simulink model "ModelWithApproximation_20210824T102023489"  (R2020a)
settings: Solver=FixedStepAuto  StartTime=0.0  StopTime=size(InputValues_20210824T100641914,1) - 1  FixedStep=1  RelTol=1e-3
model workspace (MAT data in the model file):
  InputValues_20210824T100641914 = [-5; -4.9375; -4.875; -4.8125; -4.75; -4.6875; -4.625; -4.5625; -4.5; -4.4375; -4.375; -4.3125; -4.25; -4.1875; -4.125; -4.0625; -4; -3.9375; -3.875; -3.8125; -3.75; -3.6875; -3.625; -3.5625; -3.5; -3.4375; -3.375; -3.3125; -3.25; -3.1875; -3.125; -3.0625; -3; -2.9375; -2.875; -2.8125; -2.75; -2.6875; -2.625; -2.5625; -2.5; -2.4375; -2.375; -2.3125; -2.25; -2.1875; -2.125; -2.0625; -2; -1.9375; -1.875; -1.8125; -1.75; -1.6875; -1.625; -1.5625; -1.5; -1.4375; -1.375; -1.3125; -1.25; -1.1875; -1.125; -1.0625; -1; -0.9375; -0.875; -0.8125; -0.75; -0.6875; -0.625; -0.5625; -0.5; -0.4375; -0.375; -0.3125; -0.25; -0.1875; -0.125; -0.0625; 0; 0.0625; 0.125; 0.1875; 0.25; 0.3125; 0.375; 0.4375; 0.5; 0.5625; 0.625; 0.6875; 0.75; 0.8125; 0.875; 0.9375; 1; 1.0625; 1.125; 1.1875; 1.25; 1.3125; 1.375; 1.4375; 1.5; 1.5625; 1.625; 1.6875; 1.75; 1.8125; 1.875; 1.9375; 2; 2.0625; 2.125; 2.1875; 2.25; 2.3125; 2.375; 2.4375; 2.5; 2.5625; 2.625; 2.6875; 2.75; 2.8125; 2.875; 2.9375; 3; 3.0625; 3.125; 3.1875; 3.25; 3.3125; 3.375; 3.4375; 3.5; 3.5625; 3.625; 3.6875; 3.75; 3.8125; 3.875; 3.9375; 4; 4.0625; 4.125; 4.1875; 4.25; 4.3125; 4.375; 4.4375; 4.5; 4.5625; 4.625; 4.6875; 4.75; 4.8125; 4.875; 4.9375; 5]
undefined symbols (not defined in the file or in its folder): FunctionApproximation
libraries: simulink x1
settings Model: OrderedModelArguments=off  Creator=Mahsa  LastModifiedBy=Mahsa
settings DebuggingCC: IntegerOverflowMsg=none  ParameterOverflowMsg=none  ParameterPrecisionLossMsg=none  IntegerSaturationMsg=none

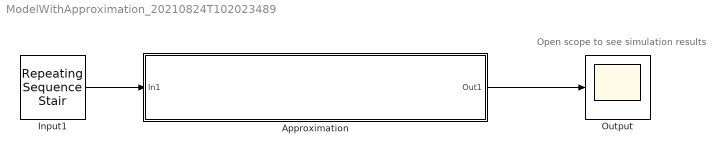
== system ModelWithApproximation_20210824T102023489 ==
  note: Open scope to see simulation results
  Approximation : Subsystem  Description=This block was created using function approximation.  Variant=on  mask(Function Approximation Solution){variantTag=3112e06394ab71adacf7bb189cb322dbc695f0e4, createdBy=FunctionApproximation, currentActive=Approximate, nApproximates=1, createdOn=20210824T102019933, matlabVersion={"Name":"MATLAB","Version":"9.8","Release":"(R2020a)","Date":"18-Nov-2019"}, functionVersion=Approximate, problemStruct={"FunctionToApproximate":"@(x)tanh(x)","InputTypes":"numerictype(1,8,4)","InputLowerBounds":"-5","InputUpperBounds":"5","OutputType":"numerictype(1,8,7)","Options":{"WordLengths":"[8]","BreakpointSpecification":"EvenPow2Spacing","AbsTol":"0.0078125","RelTol":"0.0078125","AllowUpdateDiagram":"1","Display":"0","Interpolation":"Flat","SaturateToOutputType":"1","MaxTime":"Inf","MaxMemoryUsage":"80000000","MemoryUnits":"bits","OnCurveTableValues":"0","AUTOSARCompliant":"0","UseParallel":"0"},"FunctionToReplace":"","InputFunctionType":"SpecialFunctionHandle","StorageTypes":[],"DependentVariables":[]}, compareData={"Breakpoints":[[-5,-4.9375,-4.875,-4.8125,-4.75,-4.6875,-4.625,-4.5625,-4.5,-4.4375,-4.375,-4.3125,-4.25,-4.1875,-4.125,-4.0625,-4,-3.9375,-3.875,-3.8125,-3.75,-3.6875,-3.625,-3.5625,-3.5,-3.4375,-3.375,-3.3125,-3.25,-3.1875,-3.125,-3.0625,-3,-2.9375,-2.875,-2.8125,-2.75,-2.6875,-2.625,-2.5625,-2.5,-2.4375,-2.375,-2.3125,-2.25,-2.1875,-2.125,-2.0625,-2,-1.9375,-1.875,-1.8125,-1.75,-1.6875,-1.625,-1.5625,-1.5,-1.4375,-1.375,-1.3125,-1.25,-1.1875,-1.125,-1.0625,-1,-0.9375,-0.875,-0.8125,-0.75,-0.6875,-0.625,-0.5625,-0.5,-0.4375,-0.375,-0.3125,-0.25,-0.1875,-0.125,-0.0625,0,0.0625,0.125,0.1875,0.25,0.3125,0.375,0.4375,0.5,0.5625,0.625,0.6875,0.75,0.8125,0.875,0.9375,1,1.0625,1.125,1.1875,1.25,1.3125,1.375,1.4375,1.5,1.5625,1.625,1.6875,1.75,1.8125,1.875,1.9375,2,2.0625,2.125,2.1875,2.25,2.3125,2.375,2.4375,2.5,2.5625,2.625,2.6875,2.75,2.8125,2.875,2.9375,3,3.0625,3.125,3.1875,3.25,3.3125,3.375,3.4375,3.5,3.5625,3.625,3.6875,3.75,3.8125,3.875,3.9375,4,4.0625,4.125,4.1875,4.25,4.3125,4.375,4.4375,4.5,4.5625,4.625,4.6875,4.75,4.8125,4.875,4.9375,5]],"Original":[-0.99990920426259511,-0.99989711557251559,-0.9998834174686777,-0.99986789571029067,-0.99985030754497872,-0.99983037791655283,-0.99980779516900109,-0.99978220617994684,-0.99975321084802748,-0.99972035584870533,-0.99968312756179489,-0.99964094406130644,-0.9995931460438896,-0.9995389865560137,-0.99947761936180857,-0.9994080857729738,-0.999329299739067,-0.9992400309704963,-0.99913888583735078,-0.99902428575443547,-0.9988944427261528,-0.99874733168378116,-0.99858065920179884,-0.9983918281287415,-0.99817789761119868,-0.99793553792649037,-0.997660979469889,-0.99734995516557368,-0.996997635486526,-0.99659855517712947,-0.996146530673345,-0.99563456710930964,-0.99505475368673046,-0.994398146065758,-0.99365463431502965,-0.99281279483715978,-0.9918597245682077,-0.99078085564125162,-0.98955974861288321,-0.98817786228751237,-0.98661429815143031,-0.9848455174642784,-0.982845029172576,-0.9805830470370519,-0.97802611473881362,-0.97513669829362837,-0.971872745913509,-0.96818721657637052,-0.9640275800758169,-0.95933529331468248,-0.95404526017994873,-0.9480852856044063,-0.94137553849728739,-0.93382804322259172,-0.925346225311741,-0.91582454416876236,-0.9051482536448664,-0.89319334040035159,-0.87982669965198479,-0.86490661772074184,-0.84828363995751288,-0.82980190998595948,-0.809301070201781,-0.78661881210869766,-0.76159415595576485,-0.73407151960434158,-0.70390560393662116,-0.67096707420687374,-0.6351489523872873,-0.59637355547924231,-0.55459972234938226,-0.50982997373525663,-0.46211715726000974,-0.41157005567402238,-0.35835739835078595,-0.30270972933210849,-0.24491866240370913,-0.18533319990813948,-0.12435300177159619,-0.062418746747512514,0,0.062418746747512514,0.12435300177159619,0.18533319990813948,0.24491866240370913,0.30270972933210849,0.35835739835078595,0.41157005567402238,0.46211715726000974,0.50982997373525663,0.55459972234938226,0.59637355547924231,0.6351489523872873,0.67096707420687374,0.70390560393662116,0.73407151960434158,0.76159415595576485,0.78661881210869766,0.809301070201781,0.82980190998595948,0.84828363995751288,0.86490661772074184,0.87982669965198479,0.89319334040035159,0.9051482536448664,0.91582454416876236,0.925346225311741,0.93382804322259172,0.94137553849728739,0.9480852856044063,0.95404526017994873,0.95933529331468248,0.9640275800758169,0.96818721657637052,0.971872745913509,0.97513669829362837,0.97802611473881362,0.9805830470370519,0.982845029172576,0.9848455174642784,0.98661429815143031,0.98817786228751237,0.98955974861288321,0.99078085564125162,0.9918597245682077,0.9921875,0.9921875,0.9921875,0.9921875,0.9921875,0.9921875,0.9921875,0.9921875,0.9921875,0.9921875,0.9921875,0.9921875,0.9921875,0.9921875,0.9921875,0.9921875,0.9921875,0.9921875,0.9921875,0.9921875,0.9921875,0.9921875,0.9921875,0.9921875,0.9921875,0.9921875,0.9921875,0.9921875,0.9921875,0.9921875,0.9921875,0.9921875,0.9921875,0.9921875,0.9921875,0.9921875],"Approximate":[-1,-1,-1,-1,-1,-1,-1,-1,-1,-1,-1,-1,-1,-1,-1,-1,-1,-1,-1,-1,-1,-1,-1,-1,-1,-1,-1,-1,-1,-1,-1,-0.9921875,-0.9921875,-0.9921875,-0.9921875,-0.9921875,-0.9921875,-0.9921875,-0.9921875,-0.984375,-0.984375,-0.984375,-0.984375,-0.984375,-0.9765625,-0.9765625,-0.96875,-0.96875,-0.9609375,-0.9609375,-0.953125,-0.9453125,-0.9375,-0.9375,-0.921875,-0.9140625,-0.90625,-0.890625,-0.8828125,-0.8671875,-0.8515625,-0.828125,-0.8125,-0.7890625,-0.7578125,-0.734375,-0.703125,-0.671875,-0.6328125,-0.59375,-0.5546875,-0.5078125,-0.4609375,-0.4140625,-0.359375,-0.3046875,-0.2421875,-0.1875,-0.125,-0.0625,0,0.0625,0.125,0.1875,0.2421875,0.3046875,0.359375,0.4140625,0.4609375,0.5078125,0.5546875,0.59375,0.6328125,0.671875,0.703125,0.734375,0.7578125,0.7890625,0.8125,0.828125,0.8515625,0.8671875,0.8828125,0.890625,0.90625,0.9140625,0.921875,0.9375,0.9375,0.9453125,0.953125,0.9609375,0.9609375,0.96875,0.96875,0.9765625,0.9765625,0.984375,0.984375,0.984375,0.984375,0.984375,0.9921875,0.9921875,0.9921875,0.9921875,0.9921875,0.9921875,0.9921875,0.9921875,0.9921875,0.9921875,0.9921875,0.9921875,0.9921875,0.9921875,0.9921875,0.9921875,0.9921875,0.9921875,0.9921875,0.9921875,0.9921875,0.9921875,0.9921875,0.9921875,0.9921875,0.9921875,0.9921875,0.9921875,0.9921875,0.9921875,0.9921875,0.9921875,0.9921875,0.9921875,0.9921875,0.9921875,0.9921875,0.9921875,0.9921875],"AbsDiff":[9.0795737404891774E-5,0.00010288442748440652,0.00011658253132229568,0.00013210428970933386,0.00014969245502127748,0.000169622083447174,0.00019220483099890995,0.00021779382005315817,0.00024678915197251516,0.0002796441512946668,0.00031687243820510691,0.00035905593869356434,0.00040685395611039787,0.00046101344398630228,0.0005223806381914331,0.00059191422702620233,0.000670700260932966,0.00075996902950370426,0.00086111416264922358,0.00097571424556452957,0.0011055572738472019,0.0012526683162188412,0.001419340798201163,0.0016081718712585014,0.0018221023888013166,0.002064462073509632,0.0023390205301110356,0.0026500448344263239,0.0030023645134740207,0.0034014448228705252,0.0038534693266549791,0.0034470671093096428,0.0028672536867304643,0.0022106460657580485,0.00146713431502965,0.0006252948371597844,0.00032777543179229873,0.0014066443587483768,0.0026277513871167946,0.0038028622875123652,0.0022392981514303134,0.00047051746427839714,0.0015299708274240098,0.0037919529629480975,0.0014636147388136234,0.0014258017063716322,0.0031227459135090285,0.000562783423629476,0.0030900800758169034,0.0016022066853175199,0.00092026017994872866,0.0027727856044063026,0.0038755384972873896,0.0036719567774082806,0.0034712253117410441,0.0017620441687623556,0.0011017463551336037,0.0025683404003515875,0.0029858003480152107,0.0022808822792581562,0.0032788600424871195,0.0016769099859594849,0.0031989297982190079,0.0024436878913023374,0.003781655955764851,0.00030348039565841756,0.00078060393662116034,0.000907925793126263,0.0023364523872873022,0.0026235554792423121,8.7777650617737457E-5,0.0020174737352566252,0.0011796572600097366,0.0024924443259776163,0.0010176016492140505,0.0019777706678915097,0.0027311624037091309,0.0021668000918605157,0.00064699822840380561,8.1253252487485661E-5,0,8.1253252487485661E-5,0.00064699822840380561,0.0021668000918605157,0.0027311624037091309,0.0019777706678915097,0.0010176016492140505,0.0024924443259776163,0.0011796572600097366,0.0020174737352566252,8.7777650617737457E-5,0.0026235554792423121,0.0023364523872873022,0.000907925793126263,0.00078060393662116034,0.00030348039565841756,0.003781655955764851,0.0024436878913023374,0.0031989297982190079,0.0016769099859594849,0.0032788600424871195,0.0022808822792581562,0.0029858003480152107,0.0025683404003515875,0.0011017463551336037,0.0017620441687623556,0.0034712253117410441,0.0036719567774082806,0.0038755384972873896,0.0027727856044063026,0.00092026017994872866,0.0016022066853175199,0.0030900800758169034,0.000562783423629476,0.0031227459135090285,0.0014258017063716322,0.0014636147388136234,0.0037919529629480975,0.0015299708274240098,0.00047051746427839714,0.0022392981514303134,0.0038028622875123652,0.0026277513871167946,0.0014066443587483768,0.00032777543179229873,0,0,0,0,0,0,0,0,0,0,0,0,0,0,0,0,0,0,0,0,0,0,0,0,0,0,0,0,0,0,0,0,0,0,0,0],"MaxDiff":[0.0078125,0.0078125,0.0078125,0.0078125,0.0078125,0.0078125,0.0078125,0.0078125,0.0078125,0.0078125,0.0078125,0.0078125,0.0078125,0.0078125,0.0078125,0.0078125,0.0078125,0.0078125,0.0078125,0.0078125,0.0078125,0.0078125,0.0078125,0.0078125,0.0078125,0.0078125,0.0078125,0.0078125,0.0078125,0.0078125,0.0078125,0.0078125,0.0078125,0.0078125,0.0078125,0.0078125,0.0078125,0.0078125,0.0078125,0.0078125,0.0078125,0.0078125,0.0078125,0.0078125,0.0078125,0.0078125,0.0078125,0.0078125,0.0078125,0.0078125,0.0078125,0.0078125,0.0078125,0.0078125,0.0078125,0.0078125,0.0078125,0.0078125,0.0078125,0.0078125,0.0078125,0.0078125,0.0078125,0.0078125,0.0078125,0.0078125,0.0078125,0.0078125,0.0078125,0.0078125,0.0078125,0.0078125,0.0078125,0.0078125,0.0078125,0.0078125,0.0078125,0.0078125,0.0078125,0.0078125,0.0078125,0.0078125,0.0078125,0.0078125,0.0078125,0.0078125,0.0078125,0.0078125,0.0078125,0.0078125,0.0078125,0.0078125,0.0078125,0.0078125,0.0078125,0.0078125,0.0078125,0.0078125,0.0078125,0.0078125,0.0078125,0.0078125,0.0078125,0.0078125,0.0078125,0.0078125,0.0078125,0.0078125,0.0078125,0.0078125,0.0078125,0.0078125,0.0078125,0.0078125,0.0078125,0.0078125,0.0078125,0.0078125,0.0078125,0.0078125,0.0078125,0.0078125,0.0078125,0.0078125,0.0078125,0.0078125,0.0078125,0.0078125,0.0078125,0.0078125,0.0078125,0.0078125,0.0078125,0.0078125,0.0078125,0.0078125,0.0078125,0.0078125,0.0078125,0.0078125,0.0078125,0.0078125,0.0078125,0.0078125,0.0078125,0.0078125,0.0078125,0.0078125,0.0078125,0.0078125,0.0078125,0.0078125,0.0078125,0.0078125,0.0078125,0.0078125,0.0078125,0.0078125,0.0078125,0.0078125,0.0078125],"Feasible":true,"Options":{"WordLengths":8,"BreakpointSpecification":"EvenPow2Spacing","AbsTol":0.0078125,"RelTol":0.0078125,"AllowUpdateDiagram":true,"Display":true,"Interpolation":"Flat","SaturateToOutputType":true,"MaxTime":null,"MaxMemoryUsage":8.0E+7,"MemoryUnits":"bits","OnCurveTableValues":false,"AUTOSARCompliant":false,"UseParallel":false}}}
      mask prompts: functionVersion "Select desired function version"
      mask help: This block contains the original and approximate functions.
      settings: CopyFcn=FunctionApproximation.internal.approximationblock.callback.updateTag('3112e06394ab71adacf7bb189cb322dbc695f0e4');  OpenFcn=FunctionApproximation.internal.approximationblock.callback.openMask('3112e06394ab71adacf7bb189cb322dbc695f0e4');
      mask Help: helpview(fullfile(docroot,'fixedpoint','fixedpoint.map'), 'function_approximation_block')
      mask TypeOptions functionVersion: Original | Approximate
      mask Callback functionVersion: FunctionApproximation.internal.approximationblock.callback.registerActiveFunction('3112e06394ab71adacf7bb189cb322dbc695f0e4');
      mask DialogControl details Prompt: Problem Definition
      mask DialogControl details Tooltip: Details of problem definition for approximation
      mask DialogControl detailsText Prompt:
      | Inputs for approximation:
      |   InputLowerBounds: -5
      |   InputTypes: numerictype(1,8,4)
      |   InputUpperBounds: 5
      |   OutputType: numerictype(1,8,7)
      |   Options (non-default)
      |     AbsTol: 0.0078125
      |     BreakpointSpecification: EvenPow2Spacing
      |     Display: 0
      |     Interpolation: Flat
      |     OnCurveTableValues: 0
      |     RelTol: 0.0078125
      |     SaturateToOutputType: 1
      |     WordLengths: [8]
      mask DialogControl showOriginal Prompt: Show original
      mask DialogControl showOriginal Tooltip: View the original function
      mask DialogControl showOriginal Callback: FunctionApproximation.internal.approximationblock.callback.showFunction('3112e06394ab71adacf7bb189cb322dbc695f0e4','Original');
      mask DialogControl showCurrent Prompt: Show selected
      mask DialogControl showCurrent Tooltip: View the selected function
      mask DialogControl showCurrent Callback: FunctionApproximation.internal.approximationblock.callback.showCurrent('3112e06394ab71adacf7bb189cb322dbc695f0e4');
      mask DialogControl revertToOriginal Prompt: Replace with original
      mask DialogControl revertToOriginal Tooltip: Replace current block with the original function
      mask DialogControl revertToOriginal Callback: FunctionApproximation.internal.approximationblock.callback.revertDialog('3112e06394ab71adacf7bb189cb322dbc695f0e4');
      mask DialogControl redesign Prompt: Redesign approximate
      mask DialogControl redesign Tooltip: Obtain a new approximate for the original function.
      mask DialogControl redesign Callback: FunctionApproximation.internal.approximationblock.callback.redesign('3112e06394ab71adacf7bb189cb322dbc695f0e4');
      mask DialogControl compare Prompt: Compare to original
      mask DialogControl compare Tooltip: Visualize difference between original and selected function.
      mask DialogControl compare Callback: FunctionApproximation.internal.approximationblock.callback.compareToOriginal('3112e06394ab71adacf7bb189cb322dbc695f0e4');
  Input1 : simulink/Sources/Repeating Sequence Stair  OutValues=InputValues_20210824T100641914(:,1)  tsamp=-1  OutMin=[]  OutMax=[]  OutDataTypeStr=double  OutputDataTypeScalingMode=double  OutDataType=fixdt(0,8)  ConRadixGroup=Best Precision: Vector-wise  OutScaling=2^-12
  Output : Scope
  wires:
  Input1/1 -> Approximation/1(In1)
  Approximation/1(Out1) -> Output/1

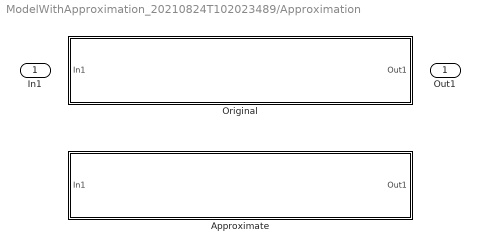
== system ModelWithApproximation_20210824T102023489/Approximation ==
  In1 : Inport
  Approximate : Subsystem  Tag=Approximate  VariantControl=FunctionApproximation.internal.approximationblock.callback.isCurrent('3112e06394ab71adacf7bb189cb322dbc695f0e4','Approximate')
  Original : Subsystem  Tag=Original  VariantControl=FunctionApproximation.internal.approximationblock.callback.isCurrent('3112e06394ab71adacf7bb189cb322dbc695f0e4','Original')
  Out1 : Outport

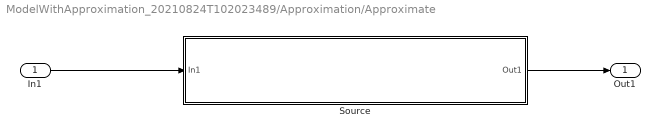
== system ModelWithApproximation_20210824T102023489/Approximation/Approximate ==
  In1 : Inport
  Source : Subsystem  Description=This block was created using function approximation.
  Out1 : Outport
  wires:
  In1/1 -> Source/1(In1)
  Source/1(Out1) -> Out1/1

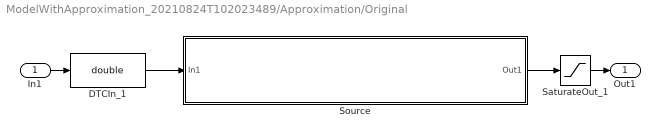
== system ModelWithApproximation_20210824T102023489/Approximation/Original ==
  In1 : Inport
  DTCIn_1 : DataTypeConversion  OutDataTypeStr=double  RndMeth=Nearest
  SaturateOut_1 : Saturate  UpperLimit=0.9921875  LowerLimit=-1
  Source : Subsystem
      mask Display: fprintf('%s','tanh')
  Out1 : Outport
  wires:
  SaturateOut_1/1 -> Out1/1
  In1/1 -> DTCIn_1/1
  DTCIn_1/1 -> Source/1(In1)
  Source/1(Out1) -> SaturateOut_1/1

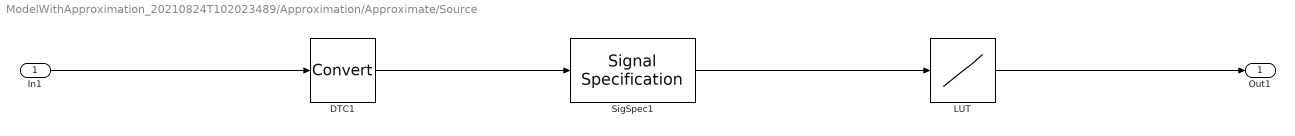
== system ModelWithApproximation_20210824T102023489/Approximation/Approximate/Source ==
  In1 : Inport
  DTC1 : DataTypeConversion  RndMeth=Nearest
  LUT : Lookup_n-D  NumberOfTableDimensions=1  LookupTableObject=FunctionApproximation_LUTObject_20210824T100641909  BreakpointsSpecification=Even spacing  BreakpointsForDimension3=[5, 7]  BreakpointsForDimension1FirstPoint=-5  BreakpointsForDimension1Spacing=0.0625  BreakpointsForDimension1DataTypeStr=numerictype(1,8,4)  IndexSearchMethod=Evenly spaced points  Table=[-1 -1 -1 -1 -1 -1 -1 -1 -1 -1 -1 -1 -1 -1 -1 -1 -1 -1 -1 -1 -1 -1 -1 -1 -1 -1 -1 -1 -1 -1 -1 -0.9921875 -0.9921875 -0.9921875 -0.9921875 -0.9921875 -0.9921875 -0.9921875 -0.9921875 -0.984375 -0.984375 -0.984375 -0.984375 -0.984375 -0.9765625 -0.9765625 -0.96875 -0.96875 -0.9609375 -0.9609375 -0.953125 -0.9453125 -0.9375 -0.9375 -0.921875 -0.9140625 -0.90625 -0.890625 -0.8828125 -0.8671875 -0.8515625 -0.828125 -0.8125 -0.7890625 -0.7578125 -0.734375 -0.703125 -0.671875 -0.6328125 -0.59375 -0.5546875 -0.5078125 -0.4609375 -0.4140625 -0.359375 -0.3046875 -0.2421875 -0.1875 -0.125 -0.0625 0 0.0625 0.125 0.1875 0.2421875 0.3046875 0.359375 0.4140625 0.4609375 0.5078125 0.5546875 0.59375 0.6328125 0.671875 0.703125 0.734375 0.7578125 0.7890625 0.8125 0.828125 0.8515625 0.8671875 0.8828125 0.890625 0.90625 0.9140625 0.921875 0.9375 0.9375 0.9453125 0.953125 0.9609375 0.9609375 0.96875 0.96875 0.9765625 0.9765625 0.984375 0.984375 0.984375 0.984375 0.984375 0.9921875 0.9921875 0.9921875 0.9921875 0.9921875 0.9921875 0.9921875 0.9921875 0.9921875 0.9921875 0.9921875 0.9921875 0.9921875 0.9921875 0.9921875 0.9921875 0.9921875 0.9921875 0.9921875 0.9921875 0.9921875 0.9921875 0.9921875 0.9921875 0.9921875 0.9921875 0.9921875 0.9921875 0.9921875 0.9921875 0.9921875 0.9921875 0.9921875 0.9921875 0.9921875 0.9921875 0.9921875]  TableDataTypeStr=numerictype(1,8,7)  InterpMethod=Flat  ExtrapMethod=Clip  UseLastTableValue=on  InternalRulePriority=Speed  OutDataTypeStr=numerictype(1,8,7)  RndMeth=Simplest  SaturateOnIntegerOverflow=on
  SigSpec1 : SignalSpecification  OutMin=-5  OutMax=5  OutDataTypeStr=numerictype(1,8,4)
  Out1 : Outport
  wires:
  LUT/1 -> Out1/1
  In1/1 -> DTC1/1
  SigSpec1/1 -> LUT/1
  DTC1/1 -> SigSpec1/1

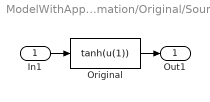
== system ModelWithApproximation_20210824T102023489/Approximation/Original/Source ==
  In1 : Inport
  Original : MATLABFcn  MATLABFcn=tanh(u(1))
  Out1 : Outport
  wires:
  In1/1 -> Original/1
  Original/1 -> Out1/1
